simulink model "vehicle_motion_model_final_temp"  (R2021b)
settings: Solver=ode5  StartTime=0.0  StopTime=600  FixedStep=0.001  RelTol=1e-3
StopFcn:
  | % stop simulation callback function
  | figure(1);
  | out.x_gt.data = permute(out.x_gt.data,[3, 1, 2]);
  | plot3(out.x_gt.data(:, 1), out.x_gt.data(:, 2), -out.x_gt.data(:, 3), 'Color', 'r', 'LineWidth', 1.5);
  | legend('Истинная траектория')
  | xlabel('X, \itм');
  | ylabel('Y, \itм');
  | zlabel('Z, \itм');
  | figure(2);
  | plot3(out.x.data(:, 1), out.x.data(:, 2), -out.x.data(:, 3), 'Color', 'b', 'LineWidth', 1.5);
  | hold on;
  | xlabel('X, \itм');
  | ylabel('Y, \itм');
  | zlabel('Z, \itм');
  | % legend('pos')
  | hold on;
  | plot3(out.x_gt.data(:, 1), out.x_gt.data(:, 2), -out.x_gt.data(:, 3), 'Color', 'r', 'LineWidth', 1.5);
  | hold on;
  | legend('Рассчитанная траектория', 'Истинная траектория')
  | % errors
  | figure(3);
  | yyaxis left;
  | plot(out.hor_err_fus.time, out.hor_err_fus.data, 'Color', 'b', 'LineWidth', 1.5);
  | xlabel('время, \itс');
  | ylabel('Горизонтальная ошибка, \itм');
  | hold on;
  | yyaxis right;
  | plot(out.ver_err_fus.time, out.ver_err_fus.data, 'Color', 'r', 'LineWidth', 1.5);
  | ylabel('Вертикальная ошибка, \itм');
  | legend('Горизонтальная позиционная ошибка', 'Вертикальная позиционная ошибка');
  | grid on;
  | figure(4);
  | yyaxis left;
  | plot(out.hor_err_ins.time, out.hor_err_ins.data, '-', 'Color', 'b', 'LineWidth', 1.5);
  | xlabel('время, \itс');
  | ylabel('Горизонтальная ошибка, \itм');
  | hold on;
  | yyaxis right;
  | plot(out.ver_err_ins.time, out.ver_err_ins.data, '-', 'Color', 'r', 'LineWidth', 1.5);
  | ylabel('Вертикальная ошибка, \itм');
  | legend('Горизонтальная позиционная ошибка', 'Вертикальная позиционная ошибка');
  | grid on;
model workspace (MAT data in the model file):
  AxlIxx = 62.3745166667
  AxlM = 160
  Cps = 2
  CzWhlAxl = 557955.087061
  DCT_Param : object (value not decoded)
  Downshift_Speeds = [9.5625 12.9375 16.3125 19.6875 23.0625 26.4375 29.8125 33.1875 36.5625 39.9375 43.3125 46.6875 ... (28 elements, 4x7)]
  F0zWhlAxl = 16132.2380068
  HTCH : object (value not decoded)
  Hmax = 0.25
  KzWhlAxl = 58428920.0848
  NCyl = 6
  Pedal_Positions = [0.1 0.4 0.5 0.9]
  Pstd = 101325
  Q = [1  0  0; 0  1  0; 0  0  1]
  Rair = 287
  SUS : object (value not decoded)
  TRA : object (value not decoded)
  Trans : object (value not decoded)
  Tstd = 293.15
  Upshift_Speeds = [12.9375 16.3125 19.6875 33 26.4375 29.8125 33.1875 52.5 39.9375 43.3125 46.6875 77.25 ... (28 elements, 4x7)]
  VEH : object (value not decoded)
  Vd = 0.00346
  WH : Mass (value not decoded)
  dt3D = 0.05
  f_air = [0 0 0 0 0 0 0 0 0 0 0 0 ... (256 elements, 16x16)]
  f_co = [0 0 0 0 0 0 0 0 0 0 0 0 ... (256 elements, 16x16)]
  f_co2 = [0 0 0 0 0 0 0 0 0 0 0 0 ... (256 elements, 16x16)]
  f_eff = [352.135682859 352.135682859 320.724378192 303.655312657 295.930136708 291.240087194 291.240271258 291.240312459 291.240275452 291.240198499 291.240100781 291.240018769 ... (256 elements, 16x16)]
  f_fuel = [0 0 0 0 0 0 0 0 0 0 0 0 ... (256 elements, 16x16)]
  f_hc = [0 0 0 0 0 0 0 0 0 0 0 0 ... (256 elements, 16x16)]
  f_nox = [0 0 0 0 0 0 0 0 0 0 0 0 ... (256 elements, 16x16)]
  f_pm = [0 0 0 0 0 0 0 0 0 0 0 0 ... (256 elements, 16x16)]
  f_susp_axl_bp = [1 2]
  f_susp_dz_bp = [-0.325022776267 -0.315022776267 -0.305022776267 -0.205022776267 -0.105022776267 -0.00502277626717 0.0949772237328 0.194977223733 0.204977223733 0.214977223733]
  f_susp_dzdot_bp = [-3 -0.3 -0.2 -0.1 0 0.1 0.2 0.3 3]
  f_susp_fmz = [-144070.391448 -93629.24037 -75929.1118915 -20630.5828179 -15385.48216 -10140.3815021 -4895.28084414 349.819813785 -31916.3973792 18437.6709544 -83996.1993354 -33555.0482577 ... (43920 elements, 10x9x61x2x4)]
  f_susp_geom = [0 0 0 0 0 0 0 0 0 0 0 0 ... (3660 elements, 10x61x2x3)]
  f_susp_strgdelta_bp = [-0.523598775598 -0.506145483078 -0.488692190558 -0.471238898038 -0.453785605519 -0.436332312999 -0.418879020479 -0.401425727959 -0.383972435439 -0.366519142919 -0.349065850399 -0.331612557879 ... (61 elements, 1x61)]
  f_tbrake = [0 76.8593923996 105.140482948 131.533638111 157.926793274 176.658631717 176.65727296 176.656856686 176.656879077 176.657093756 176.657404516 176.65772406 ... (256 elements, 16x16)]
  f_tbrake_n_bpt = [0 649.519052838 912.419621844 1175.32019085 1438.22075986 1701.12132886 1964.02189787 2226.92246687 2489.82303588 2752.72360489 3015.62417389 3278.5247429 ... (16 elements, 1x16)]
  f_tbrake_t_bpt = [0 34.6410161514 61.0341713143 87.4273264773 113.82048164 140.213636803 166.606791966 192.999947129 219.393102292 245.786257455 272.179412618 298.572567781 ... (16 elements, 1x16)]
  f_texh = [766.752464599 766.752464599 786.17542386 801.679939032 884.591982581 910.574397722 910.571871054 910.570774534 910.570601632 910.570821151 910.571247242 910.571639815 ... (256 elements, 16x16)]
  f_twc_eff_co = [0.17 0.25 0.45 0.99 0.99 0.99 0.99]
  f_twc_eff_hc = [0.21 0.375 0.75 0.98 0.98 0.98 0.98]
  f_twc_eff_lam = [0.909090909 0.944055944 0.979020979 1 1.013986014 1.048951049 1.083916084]
  f_twc_eff_nox = [0.98 0.98 0.98 0.97 0.05 0.02 0]
  h = 0.134
symbols that are objects in the model workspace (value not decoded): VEH
libraries: aerolibcommonsys x8, sharedtransform x8, sharedutil x7, autolibsharedcommon x7, autolibutils x4, vehdynlibtirecommon x3, dspstat3 x2, mspsensorlib x1, aerolibnav x1, shared6dof x1, autolibshared x1, vehdynlibsuspension x1
(part 4 of 9)

== system vehicle_motion_model_final_temp/Two-Axle Vehicle/Vehicle Body/Vehicle Body 6DOF ==
  note: modified. library link breaked
  Suspension : Inport
  Bus Selector3 : BusSelector  OutputSignals=Veh.F,Veh.M
  Constant : Constant  Value=zeros(3,1)
  Ground : Ground
  Ground1 : Ground
  Terminator{1,6..8,10..11} (6 alike) : Terminator
  Vehicle Body 6DOF : Subsystem  mask(Vehicle Body 6DOF 2 Axle){extPos=on, extVel=on, extEuler=on, extRotRate=on, htchFMode=off, htchMMode=off, m=VEH.Mass, a=VEH.FrontAxlePositionfromCG, b=VEH.RearAxlePositionfromCG, d=0, h=VEH.HeightCG, dh=VEH.HitchDistance, hl=0, hh=VEH.HitchHeight, Xe_o=[VEH.InitialLongPosition,VEH.InitialLatPosition,VEH.InitialVertPosition], xbdot_o=[VEH.InitialLongVel,VEH.InitialLatVel,VEH.InitialVertVel], eul_o=[VEH.InitialRollAngle,VEH.InitialPitchAngle,VEH.InitialYawAngle], p_o=[VEH.InitialRollRate,VEH.InitialPitchRate,VEH.InitialYawRate], Iveh=[VEH.RollMomentInertia 0 0; 0 VEH.PitchMomentInertia 0; 0 0 VEH.YawMomentInertia], w=VEH.TrackWidth.*[1 1], z1m=0, z1R=[-.25,.125,.15], z1I=[1.4,-.2,.1;-.2,1.4,.1;.1,.1,2.25].*0, z2m=0, z2R=[1.4,0,.8], z2I=[1.4,-.2,.1;-.2,1.4,.1;.1,.1,2.25].*0, z3m=0, z3R=[.75,-.5,.4], z3I=[5,-.1,-2;-2,9,.1;-.1,.1,6].*0, z4m=0, z4R=[.75,.5,.4], z4I=[5,-.1,-2;-2,9,.1;-.1,.1,6].*0, z5m=0, z5R=[1.25,-.5,.4], z5I=[5,-.1,-2;-2,9,.1;-.1,.1,6].*0, z6m=0, z6R=[1.25,-.5,.4], z6I=[5,-.1,-2;-2,9,.1;-.1,.1,6].*0, z7m=0, z7R=[2,0,.25], z7I=[1.4,-.2,.1;-.2,1.4,.1;.1,.1,2.25].*0, Af=VEH.FrontalArea, Cd=.3, Cl=.1, Cpm=.1, beta_w=[0:0.01:0.3], Cs=[0:0.03:0.9], Cym=[0:0.01:0.3], Pabs=101325, extTamb=off, Tair=273, g=9.81, xdot_tol=.1, longOff=0, latOff=0, vertOff=0.0112, wrapAng=off, aMode=2}
      mask prompts: extPos "vdynblks:vehdynVehBody6Dof:blkPrm_extPos"; extVel "vdynblks:vehdynVehBody6Dof:blkPrm_extVel"; extEuler "vdynblks:vehdynVehBody6Dof:blkPrm_extEuler"; extRotRate "vdynblks:vehdynVehBody6Dof:blkPrm_extRotRate"; htchFMode "vdynblks:vehdynVehBody6Dof:blkPrm_htchFMode"; htchMMode "vdynblks:vehdynVehBody6Dof:blkPrm_htchMMode"; m "vdynblks:vehdynVehBody6Dof:blkPrm_m"; a "vdynblks:vehdynVehBody6Dof:blkPrm_a"; b "vdynblks:vehdynVehBody6Dof:blkPrm_b"; d "vdynblks:vehdynVehBody6Dof:blkPrm_d"; h "vdynblks:vehdynVehBody6Dof:blkPrm_h"; dh "vdynblks:vehdynVehBody6Dof:blkPrm_dh"; hl "vdynblks:vehdynVehBody6Dof:blkPrm_hl"; hh "vdynblks:vehdynVehBody6Dof:blkPrm_hh"; Xe_o "vdynblks:vehdynVehBody6Dof:blkPrm_Xe_o"; xbdot_o "vdynblks:vehdynVehBody6Dof:blkPrm_xbdot_o"; eul_o "vdynblks:vehdynVehBody6Dof:blkPrm_eul_o"; p_o "vdynblks:vehdynVehBody6Dof:blkPrm_p_o"; Iveh "vdynblks:vehdynVehBody6Dof:blkPrm_Iveh"; w "vdynblks:vehdynVehBody6Dof:blkPrm_w"; z1m "vdynblks:vehdynVehBody6Dof:blkPrm_z1m"; z1R "vdynblks:vehdynVehBody6Dof:blkPrm_z1R"; z1I "vdynblks:vehdynVehBody6Dof:blkPrm_z1I"; z2m "vdynblks:vehdynVehBody6Dof:blkPrm_z2m"; z2R "vdynblks:vehdynVehBody6Dof:blkPrm_z2R"; z2I "vdynblks:vehdynVehBody6Dof:blkPrm_z2I"; z3m "vdynblks:vehdynVehBody6Dof:blkPrm_z3m"; z3R "vdynblks:vehdynVehBody6Dof:blkPrm_z3R"; z3I "vdynblks:vehdynVehBody6Dof:blkPrm_z3I"; z4m "vdynblks:vehdynVehBody6Dof:blkPrm_z4m"; z4R "vdynblks:vehdynVehBody6Dof:blkPrm_z4R"; z4I "vdynblks:vehdynVehBody6Dof:blkPrm_z4I"; z5m "vdynblks:vehdynVehBody6Dof:blkPrm_z5m"; z5R "vdynblks:vehdynVehBody6Dof:blkPrm_z5R"; z5I "vdynblks:vehdynVehBody6Dof:blkPrm_z5I"; z6m "vdynblks:vehdynVehBody6Dof:blkPrm_z6m"; z6R "vdynblks:vehdynVehBody6Dof:blkPrm_z6R"; z6I "vdynblks:vehdynVehBody6Dof:blkPrm_z6I"; z7m "vdynblks:vehdynVehBody6Dof:blkPrm_z7m"; z7R "vdynblks:vehdynVehBody6Dof:blkPrm_z7R"; z7I "vdynblks:vehdynVehBody6Dof:blkPrm_z7I"; Af "vdynblks:vehdynVehBody6Dof:blkPrm_Af"; Cd "vdynblks:vehdynVehBody6Dof:blkPrm_Cd"; Cl "vdynblks:vehdynVehBody6Dof:blkPrm_Cl"; Cpm "vdynblks:vehdynVehBody6Dof:blkPrm_Cpm"; beta_w "vdynblks:vehdynVehBody6Dof:blkPrm_beta_w"; Cs "vdynblks:vehdynVehBody6Dof:blkPrm_Cs"; Cym "vdynblks:vehdynVehBody6Dof:blkPrm_Cym"; Pabs "vdynblks:vehdynVehBody6Dof:blkPrm_Pabs"; extTamb "vdynblks:vehdynVehBody6Dof:blkPrm_extTamb"; Tair "vdynblks:vehdynVehBody6Dof:blkPrm_Tair"; g "vdynblks:vehdynVehBody6Dof:blkPrm_g"; xdot_tol "vdynblks:vehdynVehBody6Dof:blkPrm_xdot_tol"; longOff "vdynblks:vehdynVehBody6Dof:blkPrm_longOff"; latOff "vdynblks:vehdynVehBody6Dof:blkPrm_latOff"; vertOff "vdynblks:vehdynVehBody6Dof:blkPrm_vertOff"; wrapAng "vdynblks:vehdynVehBody6Dof:blkPrm_wrapAng"
      mask help: vdynblks:vehdynVehBody6Dof:blkDesc
      mask init:
      | [~] = vehdynicon('vehdynlib6dofcar',gcb,0);
      mask Help: eval('vdynblkshelp(''vb6dof'')')
      mask Callback extTamb: [~] = vehdynicon('vehdynlib6dofcar',gcb,2);
      mask DialogControl blockConfig Prompt: vdynblks:vehdynVehBody6Dof:blkDlg_blockConfig
      mask DialogControl extModePanel Prompt: vdynblks:vehdynVehBody6Dof:blkDlg_extModePanel
      mask DialogControl extPos Prompt: Position vector
      mask DialogControl extVel Prompt: Velocity vector
      mask DialogControl extEuler Prompt: Orientation vector
      mask DialogControl extRotRate Prompt: Rotation rate vector
      mask DialogControl htchFMode Prompt: Hitch forces
      mask DialogControl htchMMode Prompt: Hitch moments
      mask DialogControl vehLayoutPanel Prompt: vdynblks:vehdynVehBody6Dof:blkDlg_vehLayoutPanel
      mask DialogControl LongPanel Prompt: vdynblks:vehdynVehBody6Dof:blkDlg_LongPanel
      mask DialogControl m Prompt: Vehicle mass, m [kg]:
      mask DialogControl a Prompt: Longitudinal distance from center of mass to front axle, a [m]:
      mask DialogControl b Prompt: Longitudinal distance from center of mass to rear axle, b [m]:
      mask DialogControl d Prompt: Lateral distance from geometric centerline to center of mass, d [m]:
      mask DialogControl h Prompt: Vertical distance from center of mass to axle plane, h [m]:
      mask DialogControl dh Prompt: Longitudinal distance from center of mass to hitch, dh [m]:
      mask DialogControl hl Prompt: Lateral distance from geometric centerline to hitch, hl [m]:
      mask DialogControl hh Prompt: Vertical distance from hitch to axle plane, hh [m]:
      mask DialogControl Xe_o Prompt: Initial position in inertial frame [Xeo,Yeo,Zeo], Xe_o [m]:
      mask DialogControl xbdot_o Prompt: Initial velocity in body axes [xdot_o,ydot_o,zdot_o], xbdot_o [m/s]:
      mask DialogControl eul_o Prompt: Initial Euler orientation [roll, pitch, yaw], eul_o [rad]:
      mask DialogControl p_o Prompt: Initial body rotation rates [p,q,r], p_o [rad/s]:
      mask DialogControl Iveh Prompt: Chassis inertia tensor, Iveh [kg*m^2]:
      mask DialogControl w Prompt: Track widths [front, rear], w [m]:
      mask DialogControl loadPanel Prompt: vdynblks:vehdynVehBody6Dof:blkDlg_loadPanel
      mask DialogControl zone1Panel Prompt: vdynblks:vehdynVehBody6Dof:blkDlg_zone1Panel
      mask DialogControl z1m Prompt: Mass, z1m [kg]:
      mask DialogControl z1R Prompt: Distance vector from front axle, z1R [m]:
      mask DialogControl z1I Prompt: Inertia tensor, z1I, [kg*m^2]:
      mask DialogControl zone2Panel Prompt: vdynblks:vehdynVehBody6Dof:blkDlg_zone2Panel
      mask DialogControl z2m Prompt: Mass, z2m [kg]:
      mask DialogControl z2R Prompt: Distance vector from front axle, z2R [m]:
      mask DialogControl z2I Prompt: Inertia tensor, z2I, [kg*m^2]:
      mask DialogControl zone3Panel Prompt: vdynblks:vehdynVehBody6Dof:blkDlg_zone3Panel
      mask DialogControl z3m Prompt: Mass, z3m [kg]:
      mask DialogControl z3R Prompt: Distance vector from front axle, z3R [m]:
      mask DialogControl z3I Prompt: Inertia tensor, z3I, [kg*m^2]:
      mask DialogControl zone4Panel Prompt: vdynblks:vehdynVehBody6Dof:blkDlg_zone4Panel
      mask DialogControl z4m Prompt: Mass, z4m [kg]:
      mask DialogControl z4R Prompt: Distance vector from front axle, z4R [m]:
      mask DialogControl z4I Prompt: Inertia tensor, z4I, [kg*m^2]:
      mask DialogControl zone5Panel Prompt: vdynblks:vehdynVehBody6Dof:blkDlg_zone5Panel
      mask DialogControl z5m Prompt: Mass, z5m [kg]:
      mask DialogControl z5R Prompt: Distance vector from front axle, z5R [m]:
      mask DialogControl z5I Prompt: Inertia tensor, z5I, [kg*m^2]:
      mask DialogControl zone6Panel Prompt: vdynblks:vehdynVehBody6Dof:blkDlg_zone6Panel
      mask DialogControl z6m Prompt: Mass, z6m [kg]:
      mask DialogControl z6R Prompt: Distance vector from front axle, z6R [m]:
      mask DialogControl z6I Prompt: Inertia tensor, z6I, [kg*m^2]:
      mask DialogControl zone7Panel Prompt: vdynblks:vehdynVehBody6Dof:blkDlg_zone7Panel
      mask DialogControl z7m Prompt: Mass, z7m [kg]:
      mask DialogControl z7R Prompt: Distance vector from front axle, z7R [m]:
      mask DialogControl z7I Prompt: Inertia tensor, z7I, [kg*m^2]:
      mask DialogControl AeroParams Prompt: vdynblks:vehdynVehBody6Dof:blkDlg_AeroParams
      mask DialogControl Af Prompt: Longitudinal drag area, Af [m^2]:
      mask DialogControl Cd Prompt: Longitudinal drag coefficient, Cd [-]:
      mask DialogControl Cl Prompt: Longitudinal lift coefficient, Cl [-]:
      mask DialogControl Cpm Prompt: Longitudinal drag pitch moment, Cpm [-]:
      mask DialogControl beta_w Prompt: Relative wind angle vector, beta_w [rad]:
      mask DialogControl Cs Prompt: Side force coefficient vector, Cs [-]:
      mask DialogControl Cym Prompt: Yaw moment coefficient vector, Cym [-]:
      mask DialogControl EnviroPanel Prompt: vdynblks:vehdynVehBody6Dof:blkDlg_EnviroPanel
      mask DialogControl Pabs Prompt: Absolute Pressure, Pabs [Pa]:
      mask DialogControl extTamb Prompt: Air temperature
      mask DialogControl Tair Prompt: Air temperature, Tair [K]:
      mask DialogControl g Prompt: Gravitational acceleration, g [m/s^2]:
      mask DialogControl SimPanel Prompt: vdynblks:vehdynVehBody6Dof:blkDlg_SimPanel
      mask DialogControl xdot_tol Prompt: Longitudinal velocity tolerance, xdot_tol [m/s]:
      mask DialogControl longOff Prompt: Geometric longitudinal offset from axle plane, longOff [m]:
      mask DialogControl latOff Prompt: Geometric lateral offset from axle plane, latOff [m]:
      mask DialogControl vertOff Prompt: Geometric vertical offset from axle plane, vertOff [m]:
      mask DialogControl wrapAng Prompt: Wrap Euler angles, wrapAng
      mask Display:
      | try
      |     IconInfo = vehdynicon('vehdynlib6dofcar',gcb,8);
      | 
      |     image(IconInfo.image, IconInfo.position);
      | 
      |     for i = 1:numel(IconInfo.lconn)
      |         port_label('lconn', i, IconInfo.lconn{i})
      |     end
      | 
      |     for j = 1:numel(IconInfo.rconn)
      |         port_label('rconn', j, IconInfo.rconn{j})
      |     end
      | 
      |     for k = 1:numel(IconInfo.input)
      |         port_label('input', k, IconInfo.input{k})
      |     end
      | 
      |     for m = 1:numel(IconInfo.output)
      |         port_label('output', m, IconInfo.output{m})
      |     end
      | catch
      |     fprintf('Vehicle Body \n 6DOF Car')
      | end
  Vehicle : Outport
  wires:
  Bus Selector3/2 -> Vehicle Body 6DOF/2(MSusp)  "<M>"
  Bus Selector3/1 -> Vehicle Body 6DOF/1(FSusp)  "<F>"
  Ground/1 -> Vehicle Body 6DOF/3(FExt)
  Ground1/1 -> Vehicle Body 6DOF/4(MExt)
  Constant/1 -> Vehicle Body 6DOF/5(WindXYZ)
  Suspension/1 -> Bus Selector3/1
  Vehicle Body 6DOF/2(Vb) -> Terminator6/1
  Vehicle Body 6DOF/3(pqr) -> Terminator7/1
  Vehicle Body 6DOF/4(DCM) -> Terminator8/1
  Vehicle Body 6DOF/5(Euler) -> Terminator1/1
  Vehicle Body 6DOF/6(Xe) -> Terminator10/1
  Vehicle Body 6DOF/7(Ve) -> Terminator11/1
  Vehicle Body 6DOF/1(Info) -> Vehicle/1

== system vehicle_motion_model_final_temp/Two-Axle Vehicle/Vehicle Suspension/Steer Rate Adapter ==
  Veh : Inport
  Add : Sum
  Bus Selector3 : BusSelector  OutputSignals=BdyFrm.Cg.AngVel.r
  Constant : Constant  Value=zeros(1,4)
  Matrix Concatenate : Concatenate  NumInputs=3  Mode=Multidimensional array
  Matrix Concatenate1 : Concatenate  NumInputs=3  Mode=Multidimensional array
  Mux : Mux
  Reshape2 : Reshape  OutputDimensionality=Row vector (2-D)
  Reshape3 : Reshape  OutputDimensionality=Row vector (2-D)
  Reshape4 : Reshape  OutputDimensionality=Row vector (2-D)
  SteerRates : Constant  Value=zeros(1,4)
  AngVel : Outport  VectorParamsAs1DForOutWhenUnconnected=off
  wires:
  Reshape2/1 -> Matrix Concatenate1/1, Matrix Concatenate1/3, Matrix Concatenate1/2
  Constant/1 -> Reshape3/1
  Mux/1 -> Reshape4/1
  Bus Selector3/1 -> Mux/3, Mux/4, Mux/2, Mux/1  "<r>"
  Matrix Concatenate/1 -> Add/2
  SteerRates/1 -> Reshape2/1
  Reshape4/1 -> Matrix Concatenate/3
  Reshape3/1 -> Matrix Concatenate/2, Matrix Concatenate/1
  Matrix Concatenate1/1 -> Add/1
  Veh/1 -> Bus Selector3/1
  Add/1 -> AngVel/1  "AngVel"

== system vehicle_motion_model_final_temp/Two-Axle Vehicle/Vehicle Suspension/Steering Adapter ==
  Steer : Inport
  Reshape1 : Reshape  OutputDimensionality=Row vector (2-D)
  StrgAng : Outport  VectorParamsAs1DForOutWhenUnconnected=off
  wires:
  Reshape1/1 -> StrgAng/1
  Steer/1 -> Reshape1/1

== system vehicle_motion_model_final_temp/Two-Axle Vehicle/Vehicle Suspension/Vehicle Adapter ==
  Veh : Inport
  Bus Creator3 : BusCreator  Inputs=2
  Bus Selector1 : BusSelector  OutputSignals=InertFrm.FrntAxl.Lft.Disp.X,InertFrm.FrntAxl.Lft.Disp.Y,InertFrm.FrntAxl.Lft.Disp.Z,InertFrm.FrntAxl.Rght.Disp.X,InertFrm.FrntAxl.Rght.Disp.Y,InertFrm.FrntAxl.Rght.Disp.Z,InertFrm.RearAxl.Lft.Disp.X,InertFrm.RearAxl.Lft.Disp.Y,InertFrm.RearAxl.Lft.Disp.Z,InertFrm.RearAxl.Rght.Disp.X,InertFrm.RearAxl.Rght.Disp.Y,InertFrm.RearAxl.Rght.Disp.Z
  Bus Selector2 : BusSelector  OutputSignals=BdyFrm.FrntAxl.Lft.Vel.xdot,BdyFrm.FrntAxl.Lft.Vel.ydot,BdyFrm.FrntAxl.Lft.Vel.zdot,BdyFrm.FrntAxl.Rght.Vel.xdot,BdyFrm.FrntAxl.Rght.Vel.ydot,BdyFrm.FrntAxl.Rght.Vel.zdot,BdyFrm.RearAxl.Lft.Vel.xdot,BdyFrm.RearAxl.Lft.Vel.ydot,BdyFrm.RearAxl.Lft.Vel.zdot,BdyFrm.RearAxl.Rght.Vel.xdot,BdyFrm.RearAxl.Rght.Vel.ydot,BdyFrm.RearAxl.Rght.Vel.zdot
  Bus Selector3 : BusSelector  OutputSignals=InertFrm.FrntAxl.Lft.Vel.Xdot,InertFrm.FrntAxl.Lft.Vel.Ydot,InertFrm.FrntAxl.Lft.Vel.Zdot,InertFrm.FrntAxl.Rght.Vel.Xdot,InertFrm.FrntAxl.Rght.Vel.Ydot,InertFrm.FrntAxl.Rght.Vel.Zdot,InertFrm.RearAxl.Lft.Vel.Xdot,InertFrm.RearAxl.Lft.Vel.Ydot,InertFrm.RearAxl.Lft.Vel.Zdot,InertFrm.RearAxl.Rght.Vel.Xdot,InertFrm.RearAxl.Rght.Vel.Ydot,InertFrm.RearAxl.Rght.Vel.Zdot
  Inertial Frame CG to Axle Offset : Constant  Value=[zeros(2,4);VEH.HeightCG*ones(1,4)]
  Mux1 : Mux  Inputs=12
  Mux2 : Mux  Inputs=12
  Mux3 : Mux  Inputs=12
  Reshape : Reshape  OutputDimensionality=Customize  OutputDimensions=[3,4]
  Reshape1 : Reshape  OutputDimensionality=Customize  OutputDimensions=[3,4]
  Reshape2 : Reshape  OutputDimensionality=Customize  OutputDimensions=[3,4]
  Sum : Sum  Inputs=|+-
  VehSusp : Outport  VectorParamsAs1DForOutWhenUnconnected=off
  VehVbody : Outport  Port=2  VectorParamsAs1DForOutWhenUnconnected=off
  wires:
  Veh/1 -> Bus Selector3/1, Bus Selector2/1, Bus Selector1/1
  Reshape2/1 -> VehVbody/1  "V"
  Bus Creator3/1 -> VehSusp/1  "Veh"
  Reshape/1 -> Sum/1
  Bus Selector1/1 -> Mux2/1  "<X>"
  Bus Selector1/2 -> Mux2/2  "<Y>"
  Bus Selector1/3 -> Mux2/3  "<Z>"
  Bus Selector1/4 -> Mux2/4  "<X>"
  Bus Selector1/5 -> Mux2/5  "<Y>"
  Bus Selector1/6 -> Mux2/6  "<Z>"
  Bus Selector1/7 -> Mux2/7  "<X>"
  Bus Selector1/8 -> Mux2/8  "<Y>"
  Bus Selector1/9 -> Mux2/9  "<Z>"
  Bus Selector1/10 -> Mux2/10  "<X>"
  Bus Selector1/11 -> Mux2/11  "<Y>"
  Bus Selector1/12 -> Mux2/12  "<Z>"
  Bus Selector2/1 -> Mux1/1  "<xdot>"
  Bus Selector2/2 -> Mux1/2  "<ydot>"
  Bus Selector2/3 -> Mux1/3  "<zdot>"
  Bus Selector2/4 -> Mux1/4  "<xdot>"
  Bus Selector2/5 -> Mux1/5  "<ydot>"
  Bus Selector2/6 -> Mux1/6  "<zdot>"
  Bus Selector2/7 -> Mux1/7  "<xdot>"
  Bus Selector2/8 -> Mux1/8  "<ydot>"
  Bus Selector2/9 -> Mux1/9  "<zdot>"
  Bus Selector2/10 -> Mux1/10  "<xdot>"
  Bus Selector2/11 -> Mux1/11  "<ydot>"
  Bus Selector2/12 -> Mux1/12  "<zdot>"
  Mux1/1 -> Reshape2/1
  Mux2/1 -> Reshape/1
  Inertial Frame CG to Axle Offset/1 -> Sum/2
  Sum/1 -> Bus Creator3/1  "P"
  Mux3/1 -> Reshape1/1
  Bus Selector3/12 -> Mux3/12  "<Zdot>"
  Bus Selector3/11 -> Mux3/11  "<Ydot>"
  Bus Selector3/10 -> Mux3/10  "<Xdot>"
  Bus Selector3/9 -> Mux3/9  "<Zdot>"
  Bus Selector3/8 -> Mux3/8  "<Ydot>"
  Bus Selector3/7 -> Mux3/7  "<Xdot>"
  Bus Selector3/6 -> Mux3/6  "<Zdot>"
  Bus Selector3/5 -> Mux3/5  "<Ydot>"
  Bus Selector3/4 -> Mux3/4  "<Xdot>"
  Bus Selector3/3 -> Mux3/3  "<Zdot>"
  Bus Selector3/2 -> Mux3/2  "<Ydot>"
  Bus Selector3/1 -> Mux3/1  "<Xdot>"
  Reshape1/1 -> Bus Creator3/2  "V"

== system vehicle_motion_model_final_temp/Two-Axle Vehicle/Vehicle Suspension/Wheel  Adapter ==
  Wheels : Inport
  Bus Selector : BusSelector  OutputSignals=TireFrame.Fx,TireFrame.Fy
  Bus Selector1 : BusSelector  OutputSignals=TireFrame.Re
  Bus Selector2 : BusSelector  OutputSignals=TireFrame.Mx,TireFrame.My,TireFrame.Mz
  Bus Selector3 : BusSelector  OutputSignals=TireFrame.z,TireFrame.zdot
  Matrix Concatenate : Concatenate  NumInputs=3  Mode=Multidimensional array
  Reshape{,1..7} (8 alike) : Reshape  OutputDimensionality=Row vector (2-D)
  WhlFx : Outport  VectorParamsAs1DForOutWhenUnconnected=off
  WhlFy : Outport  Port=2  VectorParamsAs1DForOutWhenUnconnected=off
  z : Outport  Port=3  VectorParamsAs1DForOutWhenUnconnected=off
  zdot : Outport  Port=4  VectorParamsAs1DForOutWhenUnconnected=off
  M : Outport  Port=5  VectorParamsAs1DForOutWhenUnconnected=off
  Re : Outport  Port=6  VectorParamsAs1DForOutWhenUnconnected=off
  wires:
  Reshape7/1 -> WhlFy/1
  Reshape6/1 -> WhlFx/1
  Bus Selector/1 -> Reshape6/1  "<Fx>"
  Bus Selector/2 -> Reshape7/1  "<Fy>"
  Bus Selector3/1 -> Reshape/1  "<z>"
  Wheels/1 -> Bus Selector1/1, Bus Selector2/1, Bus Selector3/1, Bus Selector/1
  Bus Selector3/2 -> Reshape2/1  "<zdot>"
  Reshape2/1 -> zdot/1  "zdot"
  Bus Selector1/1 -> Reshape1/1  "<Re>"
  Reshape1/1 -> Re/1  "Re"
  Bus Selector2/1 -> Reshape3/1  "<Mx>"
  Bus Selector2/2 -> Reshape4/1  "<My>"
  Bus Selector2/3 -> Reshape5/1  "<Mz>"
  Reshape3/1 -> Matrix Concatenate/1
  Reshape4/1 -> Matrix Concatenate/2
  Reshape5/1 -> Matrix Concatenate/3
  Matrix Concatenate/1 -> M/1  "M"
  Reshape/1 -> z/1  "z"

== system vehicle_motion_model_final_temp/Two-Axle Vehicle/Vehicle Suspension/Z Force Splice ==
  note: 1) Add Subsystem or Model blocks as valid variant choices.
      | 2) You cannot connect blocks at this level. At simulation, connectivity is automatically
      | determined, based on the active variant and port name matching.
  VehFIn : Inport
  WhlFIn : Inport  Port=2
  Vehicle : Inport  Port=3
  Z Force Pass Through 6DOF : Subsystem  VariantControl=1
  Z Force Splice 3DOF : Subsystem  VariantControl=0
  VehF : Outport
  WhlF : Outport  Port=2

== system vehicle_motion_model_final_temp/Two-Axle Vehicle/Wheels and Tires/Wheels and Tires ==
  WheelAng : Inport
  CamberAng : Inport  Port=2  Unit=rad
  AxleTrq : Inport  Port=3
  BrkPrs : Inport  Port=4
  Fz : Inport  Port=5  Unit=N
  r : Inport  Port=6
  VehVel : Inport  Port=7
  Ground Level : Inport  Port=8
  Friction : Inport  Port=9  Unit=1
  Pressure : vehdynlibtirecommon/Constant  const=220000  numWheels=4
      settings: SourceProductBaseCode=VE
  Reshape : Reshape
  Terminator : Terminator
  Tire2Veh : Subsystem
  Tires : Subsystem  Variant=on  VariantControlMode=label  VariantControl=Variant1  LabelModeActiveChoice=0
  Veh2Tire : Subsystem
  scale factors with friction : Subsystem  mask{numWheels=6}
      mask prompts: numWheels "Number of wheels"
  WhlAng : Outport  VectorParamsAs1DForOutWhenUnconnected=off
  FrntAxlF : Outport  Port=2  Unit=N  VectorParamsAs1DForOutWhenUnconnected=off
  RearAxlF : Outport  Port=3  Unit=N  VectorParamsAs1DForOutWhenUnconnected=off
  Omega : Outport  Port=4  VectorParamsAs1DForOutWhenUnconnected=off
  Mz : Outport  Port=5  Unit=N*m  VectorParamsAs1DForOutWhenUnconnected=off
  SuspWhlPz : Outport  Port=6  VectorParamsAs1DForOutWhenUnconnected=off
  SuspWhlVz : Outport  Port=7  VectorParamsAs1DForOutWhenUnconnected=off
  wires:
  Ground Level/1 -> Tires/9("Gnd ")
  Pressure/1 -> Tires/7("Press ")
  scale factors with friction/1(lambdas) -> Tires/8("lambda ")
  Fz/1 -> Reshape/1
  AxleTrq/1 -> Veh2Tire/2(Axle)
  BrkPrs/1 -> Veh2Tire/3(Brake)
  VehVel/1 -> Veh2Tire/4(VehVel)
  Veh2Tire/1(T) -> Tires/1("DriveTorque ")
  Veh2Tire/2(P) -> Tires/2("Brake Pressure ")
  Veh2Tire/5(ydotAxle) -> Tires/5("Vy ")
  Veh2Tire/3(psidot) -> Tires/3("r ")
  Tires/1(" Wheels") -> Tire2Veh/1(Wheel)
  WheelAng/1 -> Veh2Tire/5(WheelSteer), Tire2Veh/4(WheelSteer)
  Tire2Veh/2(Omega) -> Omega/1
  Tire2Veh/3(FrntAxlF) -> FrntAxlF/1
  Tire2Veh/5(<Mz>) -> Mz/1
  Friction/1 -> scale factors with friction/2(lamda_mu_y), scale factors with friction/1(lamda_mu_x)
  r/1 -> Veh2Tire/1(r)
  Veh2Tire/6(zdotAxle) -> Terminator/1
  Tire2Veh/6(SuspWhlPz) -> SuspWhlPz/1
  Tire2Veh/7(SuspWhlVz) -> SuspWhlVz/1
  CamberAng/1 -> Tires/6("Camber "), Tire2Veh/3(WheelCamber), Veh2Tire/6(WheelCamber)
  Tire2Veh/1(WhlAng) -> WhlAng/1
  Tire2Veh/4(RearAxlF) -> RearAxlF/1
  Reshape/1 -> Tire2Veh/2(Fz), Tires/10("FzSusp ")
  Veh2Tire/4(xdotAxle) -> Tires/4("Vx ")

== system vehicle_motion_model_final_temp/Two-Axle Vehicle/Wheels and Tires/z forces per tire ==
  FzIn : Inport
  Demux : Demux
  Gain12 : Gain  Gain=1/VEH.NumberOfWheelsPerRearAxle
  Gain13 : Gain  Gain=1/VEH.NumberOfWheelsPerRearAxle
  Gain14 : Gain  Gain=2
  Gain8 : Gain  Gain=1/VEH.NumberOfWheelsPerFrontAxle
  Gain9 : Gain  Gain=1/VEH.NumberOfWheelsPerFrontAxle
  Mux1 : Mux
  FzTire : Outport
  wires:
  Demux/2 -> Gain9/1
  Gain14/1 -> FzTire/1
  Gain8/1 -> Mux1/1
  Mux1/1 -> Gain14/1
  Gain9/1 -> Mux1/2
  Demux/1 -> Gain8/1
  FzIn/1 -> Demux/1
  Demux/3 -> Gain12/1
  Gain12/1 -> Mux1/3
  Gain13/1 -> Mux1/4
  Demux/4 -> Gain13/1

== system vehicle_motion_model_final_temp/BINS/Three-axis Inertial Measurement Unit2/Three-axis Accelerometer/Dynamics ==
  sp_f : Inport
  Constant : Constant  Value=dtype_a
  No Dynamics : Subsystem
  Second-order Dynamics : aerolibcommonsys/Transfer Fcn (C)  wn=w_a  zn=z_a
      settings: SourceProductBaseCode=AE
  Switch : Switch  Threshold=0.5
  "sp_f " : Outport  VectorParamsAs1DForOutWhenUnconnected=off
  wires:
  sp_f/1 -> No Dynamics/1(In1), Second-order Dynamics/1
  No Dynamics/1(Out1) -> Switch/3
  Second-order Dynamics/1 -> Switch/1
  Switch/1 -> "sp_f "/1
  Constant/1 -> Switch/2

== system vehicle_motion_model_final_temp/BINS/Three-axis Inertial Measurement Unit2/Three-axis Accelerometer/w x (w x d) ==
  "p q r " : Inport
  distance : Inport  Port=2
  w x (w x d) : sharedutil/3x3 Cross Product  aMode=aMode
      settings: SourceProductBaseCode=AE,PW,DR,MT,UV,VE
  w x d : sharedutil/3x3 Cross Product  aMode=aMode
      settings: SourceProductBaseCode=AE,PW,DR,MT,UV,VE
  w x ( w x d) : Outport  VectorParamsAs1DForOutWhenUnconnected=off
  wires:
  w x (w x d)/1 -> w x ( w x d)/1
  distance/1 -> w x d/2
  w x d/1 -> w x (w x d)/2
  "p q r "/1 -> w x d/1, w x (w x d)/1

== system vehicle_motion_model_final_temp/BINS/Three-axis Inertial Measurement Unit2/Three-axis Gyroscope/Dynamics ==
  p q r : Inport
  Constant : Constant  Value=dtype_g
  No Dynamics : Subsystem
  Second-order Dynamics : aerolibcommonsys/Transfer Fcn (C)  wn=w_g  zn=z_g
      settings: SourceProductBaseCode=AE
  Switch : Switch  Threshold=0.5
  "p q r " : Outport  VectorParamsAs1DForOutWhenUnconnected=off
  wires:
  Constant/1 -> Switch/2
  Switch/1 -> "p q r "/1
  Second-order Dynamics/1 -> Switch/1
  No Dynamics/1(Out1) -> Switch/3
  p q r/1 -> No Dynamics/1(In1), Second-order Dynamics/1

== system vehicle_motion_model_final_temp/BINS/Three-axis Inertial Measurement Unit4/Three-axis Accelerometer/Dynamics ==
  sp_f : Inport
  Constant : Constant  Value=dtype_a
  No Dynamics : Subsystem
  Second-order Dynamics : aerolibcommonsys/Transfer Fcn (C)  wn=w_a  zn=z_a
      settings: SourceProductBaseCode=AE
  Switch : Switch  Threshold=0.5
  "sp_f " : Outport  VectorParamsAs1DForOutWhenUnconnected=off
  wires:
  sp_f/1 -> No Dynamics/1(In1), Second-order Dynamics/1
  No Dynamics/1(Out1) -> Switch/3
  Second-order Dynamics/1 -> Switch/1
  Switch/1 -> "sp_f "/1
  Constant/1 -> Switch/2

== system vehicle_motion_model_final_temp/BINS/Three-axis Inertial Measurement Unit4/Three-axis Accelerometer/w x (w x d) ==
  "p q r " : Inport
  distance : Inport  Port=2
  w x (w x d) : sharedutil/3x3 Cross Product  aMode=aMode
      settings: SourceProductBaseCode=AE,PW,DR,MT,UV,VE
  w x d : sharedutil/3x3 Cross Product  aMode=aMode
      settings: SourceProductBaseCode=AE,PW,DR,MT,UV,VE
  w x ( w x d) : Outport  VectorParamsAs1DForOutWhenUnconnected=off
  wires:
  w x (w x d)/1 -> w x ( w x d)/1
  distance/1 -> w x d/2
  w x d/1 -> w x (w x d)/2
  "p q r "/1 -> w x d/1, w x (w x d)/1

== system vehicle_motion_model_final_temp/BINS/Three-axis Inertial Measurement Unit4/Three-axis Gyroscope/Dynamics ==
  p q r : Inport
  Constant : Constant  Value=dtype_g
  No Dynamics : Subsystem
  Second-order Dynamics : aerolibcommonsys/Transfer Fcn (C)  wn=w_g  zn=z_g
      settings: SourceProductBaseCode=AE
  Switch : Switch  Threshold=0.5
  "p q r " : Outport  VectorParamsAs1DForOutWhenUnconnected=off
  wires:
  Constant/1 -> Switch/2
  Switch/1 -> "p q r "/1
  Second-order Dynamics/1 -> Switch/1
  No Dynamics/1(Out1) -> Switch/3
  p q r/1 -> No Dynamics/1(In1), Second-order Dynamics/1

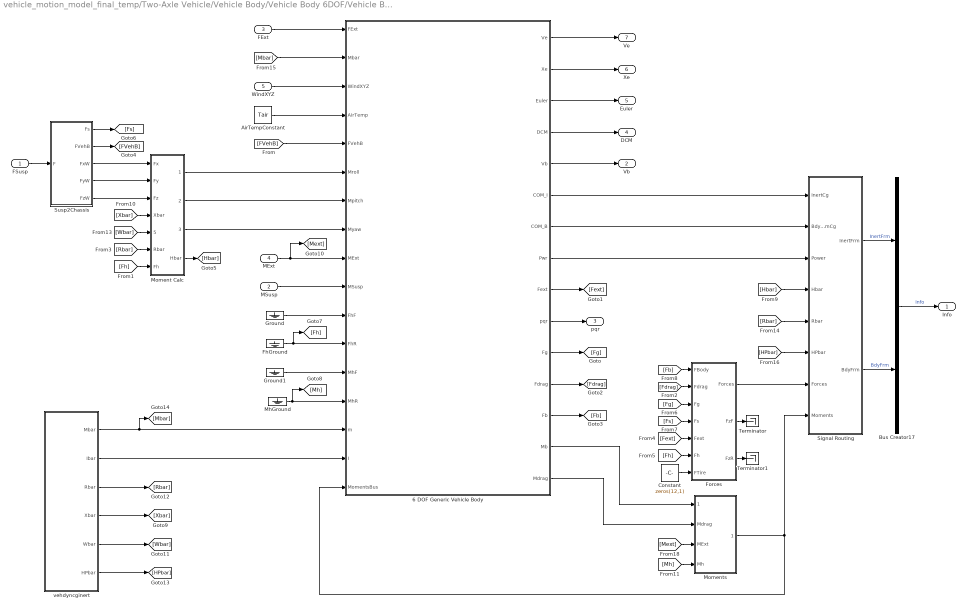
== system vehicle_motion_model_final_temp/Two-Axle Vehicle/Vehicle Body/Vehicle Body 6DOF/Vehicle Body 6DOF ==
  FSusp : Inport  Unit=N
  MSusp : Inport  Port=2  Unit=N*m
  FExt : Inport  Port=3  Unit=N
  MExt : Inport  Port=4  Unit=N*m
  WindXYZ : Inport  Port=5  Unit=m/s
  6 DOF Generic Vehicle Body : Subsystem
  AirTempConstant : Constant  Value=Tair
  Bus Creator17 : BusCreator  Inputs=2
  Constant : Constant  Value=zeros(12,1)
  FhGround : Ground
  Forces : Subsystem  VariantControl=2
  Ground : Ground
  Ground1 : Ground
  MhGround : Ground
  Moment Calc : Subsystem
  Moments : Subsystem
  Signal Routing : Subsystem  VariantControl=2
  Susp2Chassis : Subsystem
  Terminator : Terminator
  Terminator1 : Terminator
  vehdyncginert : MATLAB Function  TreatAsAtomicUnit=on
  Info : Outport  VectorParamsAs1DForOutWhenUnconnected=off
  Vb : Outport  Port=2  Unit=m/s  VectorParamsAs1DForOutWhenUnconnected=off
  pqr : Outport  Port=3  Unit=rad/s  VectorParamsAs1DForOutWhenUnconnected=off
  DCM : Outport  Port=4  VectorParamsAs1DForOutWhenUnconnected=off
  Euler : Outport  Port=5  Unit=rad  VectorParamsAs1DForOutWhenUnconnected=off
  Xe : Outport  Port=6  Unit=m  VectorParamsAs1DForOutWhenUnconnected=off
  Ve : Outport  Port=7  Unit=m/s  VectorParamsAs1DForOutWhenUnconnected=off
  wires:
  MhGround/1 -> 6 DOF Generic Vehicle Body/14(MhR), [Mh]
  Ground1/1 -> 6 DOF Generic Vehicle Body/13(MhF)
  Ground/1 -> 6 DOF Generic Vehicle Body/11(FhF)
  FhGround/1 -> 6 DOF Generic Vehicle Body/12(FhR), [Fh]
  Moments/1(Moments) -> Signal Routing/8(Moments), 6 DOF Generic Vehicle Body/17(MomentsBus)
  6 DOF Generic Vehicle Body/14(Mb) -> Moments/1(MBody)
  [Mext] -> Moments/3(MExt)
  [Mh] -> Moments/4(Mh)
  6 DOF Generic Vehicle Body/15(Mdrag) -> Moments/2(Mdrag)
  6 DOF Generic Vehicle Body/13(Fb) -> [Fb]
  6 DOF Generic Vehicle Body/12(Fdrag) -> [Fdrag]
  6 DOF Generic Vehicle Body/11(Fg) -> [Fg]
  6 DOF Generic Vehicle Body/10(pqr) -> pqr/1
  6 DOF Generic Vehicle Body/9(Fext) -> [Fext]
  6 DOF Generic Vehicle Body/8(Pwr) -> Signal Routing/3(Power)
  [Hbar] -> Signal Routing/4(Hbar)
  Moment Calc/4(Hbar) -> [Hbar]
  [Rbar] -> Moment Calc/6(Rbar)
  [Fh] -> Moment Calc/7(Fh)
  [Fh] -> Forces/6(Fh)
  Forces/1(Forces) -> Signal Routing/7(Forces)
  [FVehB] -> 6 DOF Generic Vehicle Body/5(FVehB)
  Susp2Chassis/2(FVehB) -> [FVehB]
  AirTempConstant/1 -> 6 DOF Generic Vehicle Body/4(AirTemp)
  6 DOF Generic Vehicle Body/7(COM_B) -> Signal Routing/2(BdyFrmCg)
  6 DOF Generic Vehicle Body/6(COM_I) -> Signal Routing/1(InertCg)
  6 DOF Generic Vehicle Body/5(Vb) -> Vb/1
  6 DOF Generic Vehicle Body/4(DCM) -> DCM/1
  6 DOF Generic Vehicle Body/3(Euler) -> Euler/1
  6 DOF Generic Vehicle Body/2(Xe) -> Xe/1
  6 DOF Generic Vehicle Body/1(Ve) -> Ve/1
  vehdyncginert/2(Ibar) -> 6 DOF Generic Vehicle Body/16(I)
  MSusp/1 -> 6 DOF Generic Vehicle Body/10(MSusp)
  MExt/1 -> 6 DOF Generic Vehicle Body/9(MExt), [Mext]
  Moment Calc/3(Myaw) -> 6 DOF Generic Vehicle Body/8(Myaw)
  Moment Calc/2(Mpitch) -> 6 DOF Generic Vehicle Body/7(Mpitch)
  Moment Calc/1(Mroll) -> 6 DOF Generic Vehicle Body/6(Mroll)
  WindXYZ/1 -> 6 DOF Generic Vehicle Body/3(WindXYZ)
  [Mbar] -> 6 DOF Generic Vehicle Body/2(Mbar)
  FExt/1 -> 6 DOF Generic Vehicle Body/1(FExt)
  [Rbar] -> Signal Routing/5(Rbar)
  vehdyncginert/6(HPbar) -> [HPbar]
  [HPbar] -> Signal Routing/6(HPbar)
  [Wbar] -> Moment Calc/5(Wbar)
  vehdyncginert/5(Wbar) -> [Wbar]
  vehdyncginert/4(Xbar) -> [Xbar]
  [Xbar] -> Moment Calc/4(Xbar)
  vehdyncginert/3(Rbar) -> [Rbar]
  vehdyncginert/1(Mbar) -> 6 DOF Generic Vehicle Body/15(m), [Mbar]
  Susp2Chassis/5(FzW) -> Moment Calc/3(Fz)
  Susp2Chassis/4(FyW) -> Moment Calc/2(Fy)
  Susp2Chassis/3(FxW) -> Moment Calc/1(Fx)
  [Fs] -> Forces/4(Fs)
  Forces/3(FzR) -> Terminator1/1
  Forces/2(FzF) -> Terminator/1
  Constant/1 -> Forces/7(FTire)
  [Fb] -> Forces/1(FBody)
  [Fg] -> Forces/3(Fg)
  [Fext] -> Forces/5(Fext)
  [Fdrag] -> Forces/2(Fdrag)
  Signal Routing/2(BdyFrm) -> Bus Creator17/2  "BdyFrm"
  Signal Routing/1(InertFrm) -> Bus Creator17/1  "InertFrm"
  Bus Creator17/1 -> Info/1  "Info"
  FSusp/1 -> Susp2Chassis/1(F)
  Susp2Chassis/1(Fs) -> [Fs]

== system vehicle_motion_model_final_temp/Two-Axle Vehicle/Vehicle Suspension/Z Force Splice/Z Force Pass Through 6DOF ==
  VehFIn : Inport
  WhlFIn : Inport  Port=2
  Vehicle : Inport  Port=3
  Terminator : Terminator
  VehF : Outport
  WhlF : Outport  Port=2
  wires:
  VehFIn/1 -> VehF/1  "F"
  WhlFIn/1 -> WhlF/1  "F"
  Vehicle/1 -> Terminator/1

== system vehicle_motion_model_final_temp/Two-Axle Vehicle/Vehicle Suspension/Z Force Splice/Z Force Splice 3DOF ==
  VehFIn : Inport
  WhlFIn : Inport  Port=2
  Vehicle : Inport  Port=3
  Bus Selector2 : BusSelector  OutputSignals=BdyFrm.Forces.Tires.FrntTires.Lft.Fz,BdyFrm.Forces.Tires.FrntTires.Rght.Fz,BdyFrm.Forces.Tires.RearTires.Lft.Fz,BdyFrm.Forces.Tires.RearTires.Rght.Fz
  Constant : Constant  Value=VEH.Mass*9.81/4
  Cont LPF IC : autolibutils/Cont LPF IC  wc=1/0.01  aMode=2  dataType=off
      settings: SourceProductBaseCode=PW,DR,MT,UV,VE
  Gain : Gain  Gain=-1
  Gain1 : Gain  Gain=VEH.NumberOfWheelsPerFrontAxle
  Gain2 : Gain  Gain=VEH.NumberOfWheelsPerFrontAxle
  Gain5 : Gain  Gain=VEH.NumberOfWheelsPerRearAxle
  Gain6 : Gain  Gain=VEH.NumberOfWheelsPerRearAxle
  Gain7 : Gain  Gain=1/2
  Matrix Concatenate : Concatenate  Mode=Multidimensional array
  Matrix Concatenate1 : Concatenate  Mode=Multidimensional array
  Mux : Mux
  Reshape : Reshape  OutputDimensionality=Row vector (2-D)
  Selector4 : Selector  NumberOfDimensions=2  InputPortWidth=3  IndexOptions=Index vector (dialog),Select all  Indices=[1 2],1  OutputSizes=1,1
  Selector5 : Selector  NumberOfDimensions=2  InputPortWidth=3  IndexOptions=Index vector (dialog),Select all  Indices=[1 2],1  OutputSizes=1,1
  VehF : Outport
  WhlF : Outport  Port=2
  wires:
  Vehicle/1 -> Bus Selector2/1
  Bus Selector2/4 -> Gain6/1  "<Fz>"
  Selector5/1 -> Matrix Concatenate1/1
  Gain5/1 -> Mux/3
  Constant/1 -> Cont LPF IC/2
  Matrix Concatenate/1 -> WhlF/1  "F"
  Gain1/1 -> Mux/1
  Gain7/1 -> Cont LPF IC/1
  Cont LPF IC/1 -> Reshape/1
  Gain/1 -> Matrix Concatenate1/2
  Gain2/1 -> Mux/2
  Reshape/1 -> Gain/1, Matrix Concatenate/2
  VehFIn/1 -> Selector5/1
  Selector4/1 -> Matrix Concatenate/1
  Bus Selector2/3 -> Gain5/1  "<Fz>"
  Bus Selector2/1 -> Gain1/1  "<Fz>"
  Matrix Concatenate1/1 -> VehF/1  "F"
  Mux/1 -> Gain7/1
  WhlFIn/1 -> Selector4/1
  Gain6/1 -> Mux/4
  Bus Selector2/2 -> Gain2/1  "<Fz>"

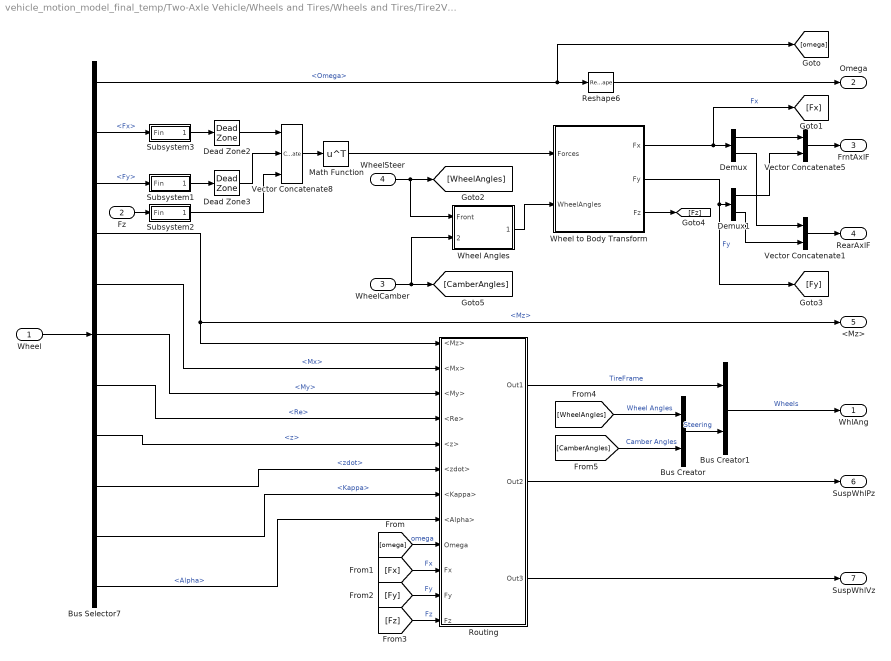
== system vehicle_motion_model_final_temp/Two-Axle Vehicle/Wheels and Tires/Wheels and Tires/Tire2Veh ==
  Wheel : Inport
  Fz : Inport  Port=2
  WheelCamber : Inport  Port=3
  WheelSteer : Inport  Port=4
  Bus Creator : BusCreator  Inputs=2
  Bus Creator1 : BusCreator  Inputs=2
  Bus Selector7 : BusSelector  OutputSignals=Omega,Fx,Fy,Mz,Mx,My,Re,z,zdot,Kappa,Alpha
  Dead Zone2 : DeadZone  LowerValue=-5  UpperValue=5  ZeroCross=off  SaturateOnIntegerOverflow=on
  Dead Zone3 : DeadZone  LowerValue=-10  UpperValue=10  ZeroCross=off  SaturateOnIntegerOverflow=on
  Demux : Demux  Outputs=[2,2]
  Demux1 : Demux  Outputs=[2,2]
  Math Function : Math  Operator=transpose  SignedPower=on  SaturateOnIntegerOverflow=on
  Reshape6 : Reshape  OutputDimensionality=Customize  OutputDimensions=[2,2]
  Routing : Subsystem
  Subsystem1 : Subsystem
  Subsystem2 : Subsystem
  Subsystem3 : Subsystem
  Vector Concatenate1 : Concatenate  Mode=Multidimensional array  ConcatenateDimension=2
  Vector Concatenate5 : Concatenate  Mode=Multidimensional array  ConcatenateDimension=2
  Vector Concatenate8 : Concatenate  NumInputs=3  Mode=Multidimensional array  ConcatenateDimension=2
  Wheel Angles : Subsystem
  Wheel to Body Transform : Subsystem
  WhlAng : Outport  VectorParamsAs1DForOutWhenUnconnected=off
  Omega : Outport  Port=2  VectorParamsAs1DForOutWhenUnconnected=off
  FrntAxlF : Outport  Port=3  VectorParamsAs1DForOutWhenUnconnected=off
  RearAxlF : Outport  Port=4  VectorParamsAs1DForOutWhenUnconnected=off
  <Mz> : Outport  Port=5  VectorParamsAs1DForOutWhenUnconnected=off
  SuspWhlPz : Outport  Port=6  VectorParamsAs1DForOutWhenUnconnected=off
  SuspWhlVz : Outport  Port=7  VectorParamsAs1DForOutWhenUnconnected=off
  wires:
  Fz/1 -> Subsystem2/1(Fin)
  Vector Concatenate8/1 -> Math Function/1
  Demux/1 -> Vector Concatenate5/1
  Math Function/1 -> Wheel to Body Transform/1(Forces)
  Dead Zone3/1 -> Vector Concatenate8/2
  Bus Selector7/2 -> Subsystem3/1(Fin)  "<Fx>"
  Dead Zone2/1 -> Vector Concatenate8/1
  Wheel to Body Transform/1(Fx) -> [Fx], Demux/1  "Fx"
  Vector Concatenate5/1 -> FrntAxlF/1
  Wheel/1 -> Bus Selector7/1
  Reshape6/1 -> Omega/1
  Demux1/1 -> Vector Concatenate5/2
  Wheel to Body Transform/2(Fy) -> Demux1/1, [Fy]  "Fy"
  Wheel Angles/1(Vehicle) -> Wheel to Body Transform/2(WheelAngles)
  Bus Selector7/1 -> [omega], Reshape6/1  "<Omega>"
  WheelSteer/1 -> Wheel Angles/1(Front), [WheelAngles]
  Bus Selector7/4 -> <Mz>/1, Routing/1(<Mz>)  "<Mz>"
  Wheel to Body Transform/3(Fz) -> [Fz]
  WheelCamber/1 -> Wheel Angles/2(Camber), [CamberAngles]
  Bus Selector7/3 -> Subsystem1/1(Fin)  "<Fy>"
  Bus Selector7/5 -> Routing/2(<Mx>)  "<Mx>"
  Bus Selector7/6 -> Routing/3(<My>)  "<My>"
  Bus Selector7/7 -> Routing/4(<Re>)  "<Re>"
  [omega] -> Routing/9(Omega)  "omega"
  [Fx] -> Routing/10(Fx)  "Fx"
  Bus Selector7/8 -> Routing/5(<z>)  "<z>"
  [Fy] -> Routing/11(Fy)  "Fy"
  [Fz] -> Routing/12(Fz)  "Fz"
  Bus Selector7/9 -> Routing/6(<zdot>)  "<zdot>"
  Bus Selector7/10 -> Routing/7(<Kappa>)  "<Kappa>"
  Routing/2(Out2) -> SuspWhlPz/1
  Routing/3(Out3) -> SuspWhlVz/1
  [WheelAngles] -> Bus Creator/1  "Wheel Angles"
  Bus Creator1/1 -> WhlAng/1  "Wheels"
  Routing/1(Out1) -> Bus Creator1/1  "TireFrame"
  [CamberAngles] -> Bus Creator/2  "Camber Angles"
  Bus Creator/1 -> Bus Creator1/2  "Steering"
  Bus Selector7/11 -> Routing/8(<Alpha>)  "<Alpha>"
  Vector Concatenate1/1 -> RearAxlF/1
  Demux/2 -> Vector Concatenate1/1
  Demux1/2 -> Vector Concatenate1/2
  Subsystem2/1(Fout) -> Vector Concatenate8/3
  Subsystem1/1(Fout) -> Dead Zone3/1
  Subsystem3/1(Fout) -> Dead Zone2/1

== system vehicle_motion_model_final_temp/Two-Axle Vehicle/Wheels and Tires/Wheels and Tires/Tires ==
  "DriveTorque " : Inport
  "Brake Pressure " : Inport  Port=2
  "r " : Inport  Port=3
  "Vx " : Inport  Port=4
  "Vy " : Inport  Port=5
  "Camber " : Inport  Port=6
  "Press " : Inport  Port=7
  "lambda " : Inport  Port=8
  "Gnd " : Inport  Port=9
  "FzSusp " : Inport  Port=10
  Fiala Tires : Subsystem  VariantControl=1
  MF Tires : Subsystem  VariantControl=0
  " Wheels" : Outport  VectorParamsAs1DForOutWhenUnconnected=off

== system vehicle_motion_model_final_temp/Two-Axle Vehicle/Wheels and Tires/Wheels and Tires/Veh2Tire ==
  r : Inport
  Axle : Inport  Port=2
  Brake : Inport  Port=3
  VehVel : Inport  Port=4
  WheelSteer : Inport  Port=5
  WheelCamber : Inport  Port=6
  Demux4 : Demux
  Gain4 : Gain  Gain=[1;-1;1;-1]*0+1
  Mux1 : Mux
  Reshape3 : Reshape
  Reshape4 : Reshape
  Unary Minus : UnaryMinus
  Wheel Angles : Subsystem
  Wheel to Body Transform : Subsystem
  T : Outport  Unit=N*m  VectorParamsAs1DForOutWhenUnconnected=off
  P : Outport  Port=2  Unit=Pa  VectorParamsAs1DForOutWhenUnconnected=off
  psidot : Outport  Port=3  Unit=rad/s  VectorParamsAs1DForOutWhenUnconnected=off
  xdotAxle : Outport  Port=4  Unit=m/s  VectorParamsAs1DForOutWhenUnconnected=off
  ydotAxle : Outport  Port=5  Unit=m/s  VectorParamsAs1DForOutWhenUnconnected=off
  zdotAxle : Outport  Port=6  Unit=m/s  VectorParamsAs1DForOutWhenUnconnected=off
  wires:
  Brake/1 -> Reshape3/1
  Axle/1 -> Reshape4/1
  Wheel to Body Transform/1(xdotWheel) -> xdotAxle/1  "Vx"
  Wheel to Body Transform/2(ydotWheel) -> ydotAxle/1  "Vy"
  WheelSteer/1 -> Wheel Angles/1(steer)
  Mux1/1 -> P/1
  r/1 -> Unary Minus/1
  Reshape3/1 -> Demux4/1
  Gain4/1 -> T/1
  Reshape4/1 -> Gain4/1
  VehVel/1 -> Wheel to Body Transform/1(VelVeh)
  Wheel to Body Transform/3(zdotWheel) -> zdotAxle/1  "Vz"
  WheelCamber/1 -> Wheel Angles/2(camber)
  Unary Minus/1 -> psidot/1
  Wheel Angles/1(Vehicle) -> Wheel to Body Transform/2(WheelAngles)
  Demux4/1 -> Mux1/1
  Demux4/2 -> Mux1/2
  Demux4/3 -> Mux1/3
  Demux4/4 -> Mux1/4

== system vehicle_motion_model_final_temp/Two-Axle Vehicle/Wheels and Tires/Wheels and Tires/scale factors with friction ==
  lamda_mu_x : Inport
  lamda_mu_y : Inport  Port=2
  0 : Constant  Value=[zeros(1,4)]  VectorParams1D=off
  Reshape : Reshape  OutputDimensionality=Row vector (2-D)  OutputDimensions=[1,numWheels]
  Reshape1 : Reshape  OutputDimensionality=Row vector (2-D)  OutputDimensions=[1,numWheels]
  Signal Specification3 : SignalSpecification  Unit=1
  Vector Concatenate : Concatenate  NumInputs=5  Mode=Multidimensional array
  ones : Constant  Value=[ones(23,4)]  VectorParams1D=off
  ones2 : Constant  Value=ones(1,4)  VectorParams1D=off
  lambdas : Outport  Unit=1  VectorParamsAs1DForOutWhenUnconnected=off
  wires:
  lamda_mu_y/1 -> Reshape1/1
  lamda_mu_x/1 -> Reshape/1
  ones2/1 -> Vector Concatenate/1  "lambda_Fz0"
  Vector Concatenate/1 -> Signal Specification3/1
  ones/1 -> Vector Concatenate/5
  0/1 -> Vector Concatenate/4  "lamda_mu_V"
  Reshape1/1 -> Vector Concatenate/3
  Reshape/1 -> Vector Concatenate/2
  Signal Specification3/1 -> lambdas/1

== system vehicle_motion_model_final_temp/BINS/Three-axis Inertial Measurement Unit2/Three-axis Accelerometer/Dynamics/No Dynamics ==
  In1 : Inport
  Out1 : Outport  VectorParamsAs1DForOutWhenUnconnected=off
  wires:
  In1/1 -> Out1/1

== system vehicle_motion_model_final_temp/BINS/Three-axis Inertial Measurement Unit2/Three-axis Gyroscope/Dynamics/No Dynamics ==
  In1 : Inport
  Out1 : Outport  VectorParamsAs1DForOutWhenUnconnected=off
  wires:
  In1/1 -> Out1/1

== system vehicle_motion_model_final_temp/BINS/Three-axis Inertial Measurement Unit4/Three-axis Accelerometer/Dynamics/No Dynamics ==
  In1 : Inport
  Out1 : Outport  VectorParamsAs1DForOutWhenUnconnected=off
  wires:
  In1/1 -> Out1/1

== system vehicle_motion_model_final_temp/BINS/Three-axis Inertial Measurement Unit4/Three-axis Gyroscope/Dynamics/No Dynamics ==
  In1 : Inport
  Out1 : Outport  VectorParamsAs1DForOutWhenUnconnected=off
  wires:
  In1/1 -> Out1/1
